simulink model "MDM_v2"  (R2018b)
settings: Solver=VariableStepAuto  StartTime=0.0  StopTime=10.0  RelTol=1e-3
undefined symbols (not defined in the file): C2, Cs, Cwc, I3, I4, I5, Ie, Jr, Jt, Jw, k1, k2, k3, k4, k5, k8, Mt, R5, Rb, Re, Rg, Rs, Rwc
settings Model: Creator=HYJ  LastModifiedBy=HYJ

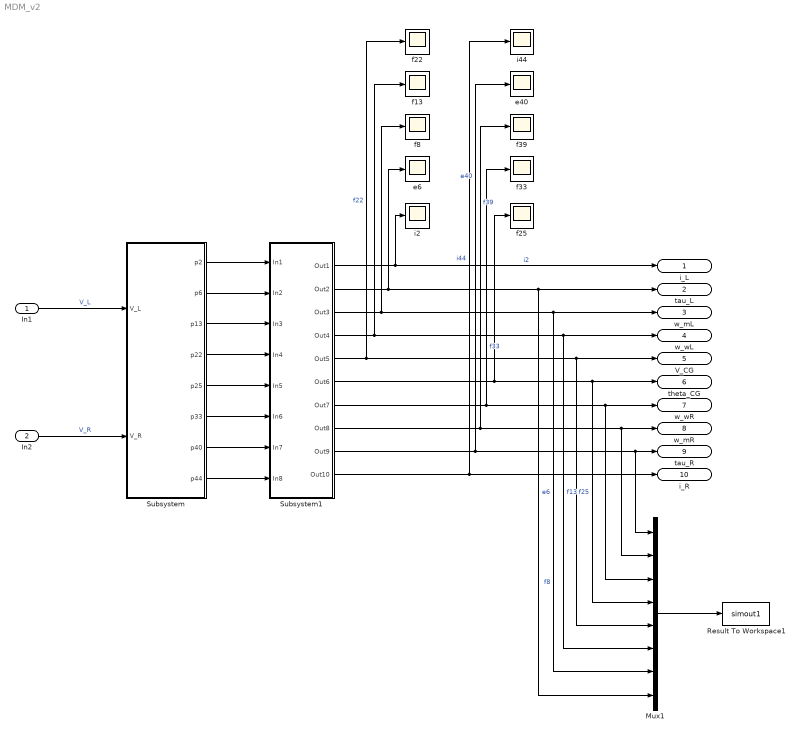
== system MDM_v2 ==
  In1 : Inport
  In2 : Inport  Port=2
  Mux1 : Mux  Inputs=8
  Result To Workspace1 : ToWorkspace  VariableName=simout1  SaveFormat=Timeseries  SampleTime=-1
  Subsystem : Subsystem
  Subsystem1 : Subsystem
  e40 : Scope
  e6 : Scope
  f{8,13,22,25,33,39} (6 alike) : Scope
  i2 : Scope
  i44 : Scope
  i_L : Outport
  tau_L : Outport  Port=2
  w_mL : Outport  Port=3
  w_wL : Outport  Port=4
  V_CG : Outport  Port=5
  theta_CG : Outport  Port=6
  w_wR : Outport  Port=7
  w_mR : Outport  Port=8
  tau_R : Outport  Port=9
  i_R : Outport  Port=10
  wires:
  In1/1 -> Subsystem/1(V_L)  "V_L"
  In2/1 -> Subsystem/2(V_R)  "V_R"
  Mux1/1 -> Result To Workspace1/1
  Subsystem/1(p2) -> Subsystem1/1(In1)
  Subsystem/2(p6) -> Subsystem1/2(In2)
  Subsystem/3(p13) -> Subsystem1/3(In3)
  Subsystem/4(p22) -> Subsystem1/4(In4)
  Subsystem/5(p25) -> Subsystem1/5(In5)
  Subsystem/6(p33) -> Subsystem1/6(In6)
  Subsystem/7(p40) -> Subsystem1/7(In7)
  Subsystem/8(p44) -> Subsystem1/8(In8)
  Subsystem1/1(Out1) -> i2/1, i_L/1  "i2"
  Subsystem1/2(Out2) -> e6/1, Mux1/8, tau_L/1  "e6"
  Subsystem1/3(Out3) -> f8/1, Mux1/7, w_mL/1  "f8"
  Subsystem1/4(Out4) -> f13/1, Mux1/6, w_wL/1  "f13"
  Subsystem1/5(Out5) -> f22/1, Mux1/5, V_CG/1  "f22"
  Subsystem1/6(Out6) -> f25/1, Mux1/4, theta_CG/1  "f25"
  Subsystem1/7(Out7) -> Mux1/3, w_wR/1, f33/1  "f33"
  Subsystem1/8(Out8) -> f39/1, Mux1/2, w_mR/1  "f39"
  Subsystem1/9(Out9) -> e40/1, Mux1/1, tau_R/1  "e40"
  Subsystem1/10(Out10) -> i44/1, i_R/1  "i44"

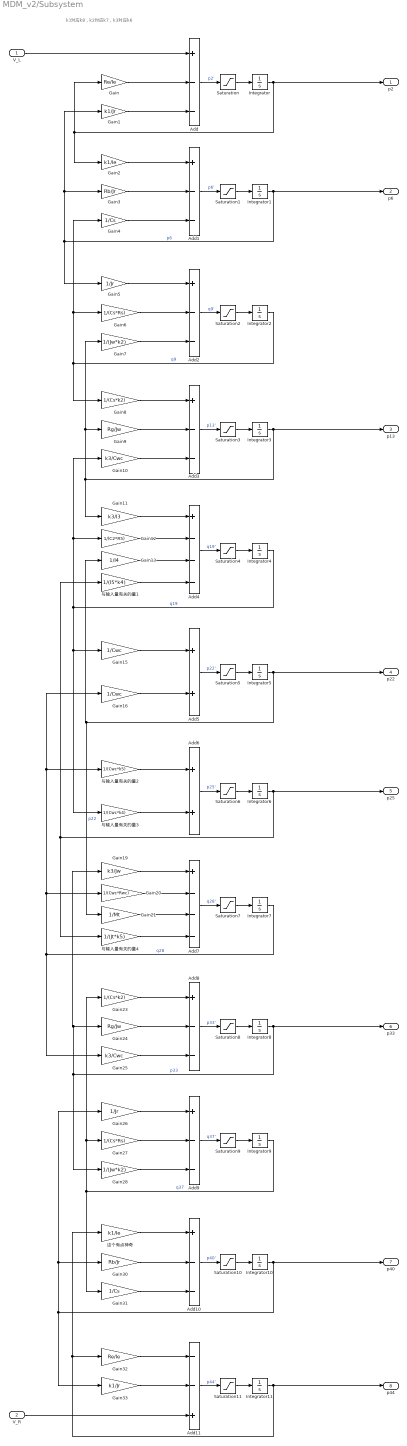
== system MDM_v2/Subsystem ==
  note: k1对应k8，k2对应k7，k3对应k6
  V_L : Inport
  V_R : Inport  Port=2
  Add{,1..3,8..10} (7 alike) : Sum  Inputs=+--
  Add11 : Sum  Inputs=--+
  Add4 : Sum  Inputs=+---
  Add5 : Sum
  Add6 : Sum
  Add7 : Sum  Inputs=+---
  Gain : Gain  Gain=Re/Ie
  Gain1 : Gain  Gain=k1/Jr
  Gain10 : Gain  Gain=k3/Cwc
  Gain11 : Gain  Gain=k3/I3
  Gain12 : Gain  Gain=1/(C2*R5)
  Gain13 : Gain  Gain=1/I4
  Gain15 : Gain  Gain=1/Cwc
  Gain16 : Gain  Gain=1/Cwc
  Gain19 : Gain  Gain=k3/Jw
  Gain2 : Gain  Gain=k1/Ie
  Gain20 : Gain  Gain=1/(Cwc*Rwc)
  Gain21 : Gain  Gain=1/Mt
  Gain23 : Gain  Gain=1/(Cs*k2)
  Gain24 : Gain  Gain=Rg/Jw
  Gain25 : Gain  Gain=k3/Cwc
  Gain26 : Gain  Gain=1/Jr
  Gain27 : Gain  Gain=1/(Cs*Rs)
  Gain28 : Gain  Gain=1/(Jw*k2)
  Gain3 : Gain  Gain=Rb/Jr
  Gain30 : Gain  Gain=Rb/Jr
  Gain31 : Gain  Gain=1/Cs
  Gain32 : Gain  Gain=Re/Ie
  Gain33 : Gain  Gain=k1/Jr
  Gain4 : Gain  Gain=1/Cs
  Gain5 : Gain  Gain=1/Jr
  Gain6 : Gain  Gain=1/(Cs*Rs)
  Gain7 : Gain  Gain=1/(Jw*k2)
  Gain8 : Gain  Gain=1/(Cs*k2)
  Gain9 : Gain  Gain=Rg/Jw
  Integrator{,1..11} (12 alike) : Integrator
  Saturation{,1..11} (12 alike) : Saturate  UpperLimit=100  LowerLimit=-100
  与输入量有关的量1 : Gain  Gain=1/(I5*k4)
  与输入量有关的量2 : Gain  Gain=1/(Cwc*k5)
  与输入量有关的量3 : Gain  Gain=1/(Cwc*k4)
  与输入量有关的量4 : Gain  Gain=1/(Jt*k5)
  这个有点神奇 : Gain  Gain=k1/Ie
  p2 : Outport
  p6 : Outport  Port=2
  p13 : Outport  Port=3
  p22 : Outport  Port=4
  p25 : Outport  Port=5
  p33 : Outport  Port=6
  p40 : Outport  Port=7
  p44 : Outport  Port=8
  wires:
  Add3/1 -> Saturation3/1  "p13'"
  Gain9/1 -> Add3/2
  Integrator5/1 -> p22/1, Gain21/1, Gain13/1  "p22"
  Add10/1 -> Saturation10/1  "p40'"
  Saturation/1 -> Integrator/1
  Gain13/1 -> Add4/3
  Integrator/1 -> p2/1, Gain2/1, Gain/1
  Saturation1/1 -> Integrator1/1
  Gain32/1 -> Add11/1
  Gain1/1 -> Add/3
  Gain26/1 -> Add9/1
  Add1/1 -> Saturation1/1  "p6'"
  Gain3/1 -> Add1/2
  Gain2/1 -> Add1/1
  Integrator7/1 -> Gain25/1, Gain20/1, Gain16/1, 与输入量有关的量2/1  "q28"
  Gain7/1 -> Add2/3
  Integrator1/1 -> p6/1, Gain5/1, Gain3/1, Gain1/1  "p6"
  Integrator2/1 -> Gain4/1, Gain6/1, Gain8/1  "q9"
  Gain6/1 -> Add2/2
  Saturation2/1 -> Integrator2/1
  Gain16/1 -> Add5/2
  Gain15/1 -> Add5/1
  Saturation5/1 -> Integrator5/1
  Add2/1 -> Saturation2/1  "q9'"
  Add/1 -> Saturation/1  "p2'"
  Saturation7/1 -> Integrator7/1
  Saturation6/1 -> Integrator6/1
  Gain21/1 -> Add7/3
  Integrator4/1 -> 与输入量有关的量3/1, Gain15/1, Gain12/1, Gain10/1  "q19"
  Add4/1 -> Saturation4/1  "q19'"
  与输入量有关的量1/1 -> Add4/4
  Integrator8/1 -> p33/1, Gain28/1, Gain24/1, Gain19/1  "p33"
  Add6/1 -> Saturation6/1  "p25'"
  Add5/1 -> Saturation5/1  "p22'"
  Integrator10/1 -> p40/1, Gain33/1, Gain26/1, Gain30/1
  Integrator3/1 -> p13/1, Gain9/1, Gain7/1, Gain11/1
  Integrator6/1 -> p25/1, 与输入量有关的量4/1, 与输入量有关的量1/1
  Saturation4/1 -> Integrator4/1
  Saturation3/1 -> Integrator3/1
  Gain30/1 -> Add10/2
  与输入量有关的量3/1 -> Add6/2
  Add7/1 -> Saturation7/1  "q28'"
  Gain20/1 -> Add7/2
  Gain33/1 -> Add11/2
  Gain5/1 -> Add2/1
  Integrator9/1 -> Gain31/1, Gain23/1, Gain27/1  "q37"
  Gain23/1 -> Add8/1
  Gain10/1 -> Add3/3
  Gain11/1 -> Add4/1
  Gain19/1 -> Add7/1
  Saturation11/1 -> Integrator11/1
  Gain8/1 -> Add3/1
  Gain27/1 -> Add9/2
  这个有点神奇/1 -> Add10/1
  Gain/1 -> Add/2
  Add9/1 -> Saturation9/1  "q37'"
  Saturation9/1 -> Integrator9/1
  Gain28/1 -> Add9/3
  Gain25/1 -> Add8/3
  Add8/1 -> Saturation8/1  "p33'"
  与输入量有关的量2/1 -> Add6/1
  Add11/1 -> Saturation11/1  "p44'"
  与输入量有关的量4/1 -> Add7/4
  Gain12/1 -> Add4/2
  Gain31/1 -> Add10/3
  Gain24/1 -> Add8/2
  Saturation10/1 -> Integrator10/1
  Saturation8/1 -> Integrator8/1
  Integrator11/1 -> p44/1, 这个有点神奇/1, Gain32/1
  Gain4/1 -> Add1/3
  V_L/1 -> Add/1
  V_R/1 -> Add11/3

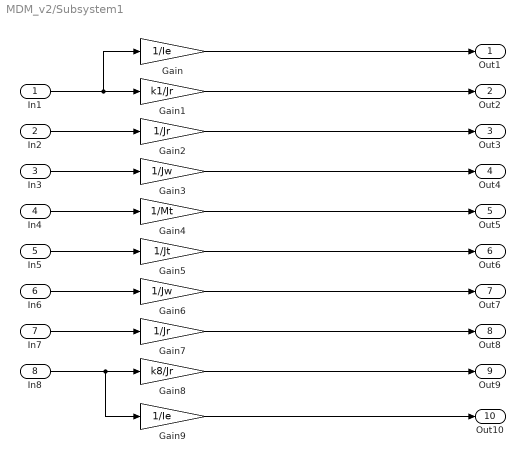
== system MDM_v2/Subsystem1 ==
  In1 : Inport
  In2 : Inport  Port=2
  In3 : Inport  Port=3
  In4 : Inport  Port=4
  In5 : Inport  Port=5
  In6 : Inport  Port=6
  In7 : Inport  Port=7
  In8 : Inport  Port=8
  Gain : Gain  Gain=1/Ie
  Gain1 : Gain  Gain=k1/Jr
  Gain2 : Gain  Gain=1/Jr
  Gain3 : Gain  Gain=1/Jw
  Gain4 : Gain  Gain=1/Mt
  Gain5 : Gain  Gain=1/Jt
  Gain6 : Gain  Gain=1/Jw
  Gain7 : Gain  Gain=1/Jr
  Gain8 : Gain  Gain=k8/Jr
  Gain9 : Gain  Gain=1/Ie
  Out1 : Outport
  Out2 : Outport  Port=2
  Out3 : Outport  Port=3
  Out4 : Outport  Port=4
  Out5 : Outport  Port=5
  Out6 : Outport  Port=6
  Out7 : Outport  Port=7
  Out8 : Outport  Port=8
  Out9 : Outport  Port=9
  Out10 : Outport  Port=10
  wires:
  In7/1 -> Gain7/1
  In1/1 -> Gain/1, Gain1/1
  Gain8/1 -> Out9/1
  Gain/1 -> Out1/1
  In8/1 -> Gain9/1, Gain8/1
  Gain3/1 -> Out4/1
  Gain1/1 -> Out2/1
  Gain6/1 -> Out7/1
  Gain5/1 -> Out6/1
  Gain2/1 -> Out3/1
  Gain7/1 -> Out8/1
  In5/1 -> Gain5/1
  In4/1 -> Gain4/1
  In6/1 -> Gain6/1
  In2/1 -> Gain2/1
  In3/1 -> Gain3/1
  Gain9/1 -> Out10/1
  Gain4/1 -> Out5/1
